simulink model "Model_OnlyDark_17_01_16"  (R2015a)
settings: Solver=FixedStepDiscrete  StartTime=0.0  StopTime=60  FixedStep=0.05  RelTol=1e-3
InitFcn:
  | %Ts=parameter.Ts;
  |    %Sampling Time, 50 times slower than original model
model workspace (MAT data in the model file):
  TimeStep = 0.05
  padsize = 8
  x1 = 14
  pixPR = 12
  hdegs = 90
  vdegs = 20
undefined symbols (not defined in the file): alpha_downslope_off, alpha_downslope_on, alpha_upslope_off, alpha_upslope_on, fdsr_lp
libraries: visionfilter x3, visionutilities x3
settings Model: tstep=0.1  TimeStep=0.1  CovSFcnEnable=off  Creator=a1174239  LastModifiedBy=John
settings SolverCC: AlgebraicLoopSolver=LineSearch
settings DataIOCC: MaxDataPoints=1
settings OptimizationCC: ExpressionDepthLimit=2147483647  EfficientMapNaN2IntZero=off
settings DebuggingCC: UnderspecifiedInitializationDetection=Classic  MergeDetectMultiDrivingBlocksExec=none  SolverPrmCheckMsg=warning  MultiTaskDSMMsg=warning  MultiTaskCondExecSysMsg=none  ParameterPrecisionLossMsg=none  StateNameClashWarn=warning
settings HardwareCC: TargetLongLongMode=on  TargetIntDivRoundTo=Zero  TargetEndianess=LittleEndian  TargetHWDeviceType=MATLAB Host  ProdEqTarget=off
settings CodeAppCC: MaxIdLength=128
settings GRTTargetCC: CombineOutputUpdateFcns=off  GRTInterface=on

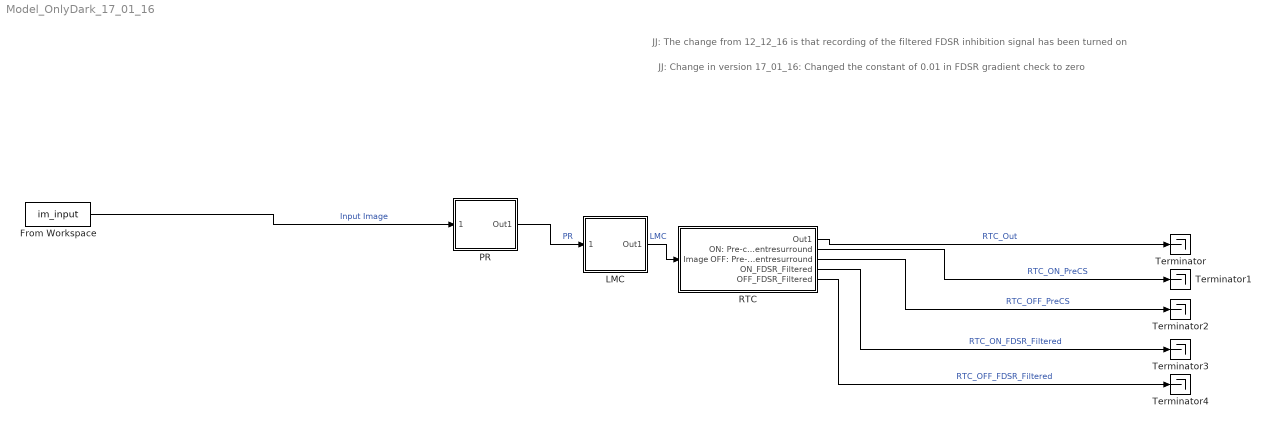
== system Model_OnlyDark_17_01_16 ==
  note: JJ: Change in version 17_01_16: Changed the constant of 0.01 in FDSR gradient check to zero
  note: JJ: The change from 12_12_16 is that recording of the filtered FDSR inhibition signal has been turned on
  From Workspace : FromWorkspace  VariableName=im_input  SampleTime=0.001  Interpolate=off  OutputAfterFinalValue=Holding final value
  LMC : Subsystem
  PR : Subsystem
  RTC : Subsystem
  Terminator{,1..4} (5 alike) : Terminator
  wires:
  PR/1(Out1) -> LMC/1(Image)  "PR"
  LMC/1(Out1) -> RTC/1(Image)  "LMC"
  RTC/1(Out1) -> Terminator/1  "RTC_Out"
  From Workspace/1 -> PR/1(Image)  "Input Image"
  RTC/2(ON: Pre-centresurround) -> Terminator1/1  "RTC_ON_PreCS"
  RTC/3(OFF: Pre-centresurround) -> Terminator2/1  "RTC_OFF_PreCS"
  RTC/4(ON_FDSR_Filtered) -> Terminator3/1  "RTC_ON_FDSR_Filtered"
  RTC/5(OFF_FDSR_Filtered) -> Terminator4/1  "RTC_OFF_FDSR_Filtered"

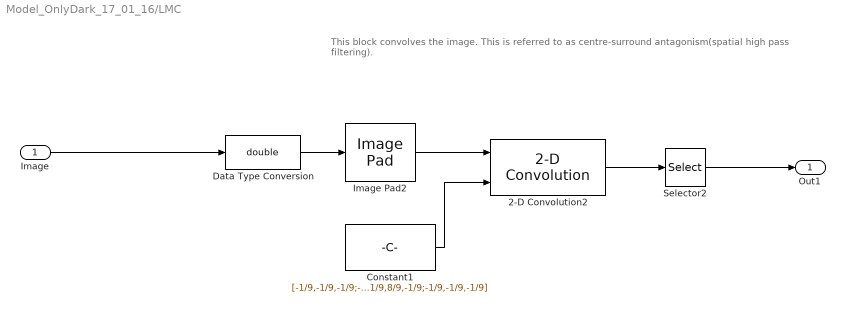
== system Model_OnlyDark_17_01_16/LMC ==
  note: This block convolves the image. This is referred to as centre-surround antagonism(spatial high pass filtering).
  Image : Inport
  2-D Convolution2 : visionfilter/2-D Convolution  outSize=Same as input port I1  normalize=off  outputMode=Binary point scaling  outputWordLength=32  outputFracLength=12  prodOutputMode=Binary point scaling  prodOutputWordLength=32  prodOutputFracLength=10  roundingMode=Floor  overflowMode=off
  Constant1 : Constant  Value=[-1/9,-1/9,-1/9;-1/9,8/9,-1/9;-1/9,-1/9,-1/9]
  Data Type Conversion : DataTypeConversion  OutDataTypeStr=double
  Image Pad2 : visionutilities/Image Pad  method=Symmetric  valSrc=Specify via dialog  value=0  spec=Pad size  rowDirection=Both left and right  outRowsMode=User-specified  rowSize=1  outColSize=10  colDirection=Both top and bottom  outColsMode=User-specified  colSize=1  outRowSize=12  trunc_flag=None
  Selector2 : Selector  NumberOfDimensions=2  InputPortWidth=3  IndexOptions=Index vector (dialog),Index vector (dialog)  Indices=[2:vdegs+1],[2:hdegs+1]  OutputSizes=1,1
  Out1 : Outport
  wires:
  Constant1/1 -> 2-D Convolution2/2
  Image Pad2/1 -> 2-D Convolution2/1
  2-D Convolution2/1 -> Selector2/1
  Selector2/1 -> Out1/1
  Image/1 -> Data Type Conversion/1
  Data Type Conversion/1 -> Image Pad2/1

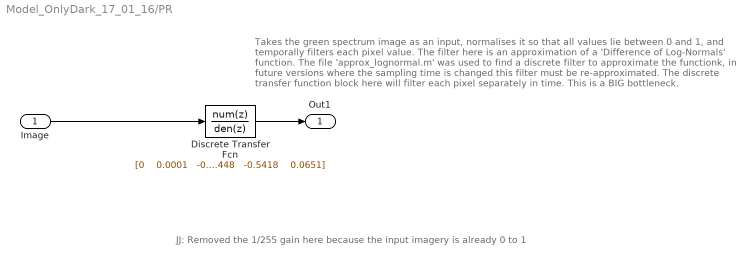
== system Model_OnlyDark_17_01_16/PR ==
  note: JJ: Removed the 1/255 gain here because the input imagery is already 0 to 1
  note: Takes the green spectrum image as an input, normalises it so that all values lie between 0
      | and 1, and temporally filters each pixel value. The filter here is an approximation of a
      | 'Difference of Log-Normals' function. The file 'approx_lognormal.m' was used to find a discrete
      | filter to approximate the functionk, in future versions where the sampling time is changed this filter
      | must be re-approximated.
      |
      | The discrete transfer function block here will filter each pixel separately in time. This is a BIG bottleneck.
  Image : Inport
  Discrete Transfer Fcn : DiscreteTransferFcn  Numerator="[0    0.0001   -0.0011    0.0052   -0.0170    0.0439   -0.0574    0.1789   -0.1524]"  Denominator="[ 1.0000   -4.3331    8.6847  -10.7116    9.0004   -5.3058    2.1448   -0.5418    0.0651]"
  Out1 : Outport
  wires:
  Image/1 -> Discrete Transfer Fcn/1
  Discrete Transfer Fcn/1 -> Out1/1

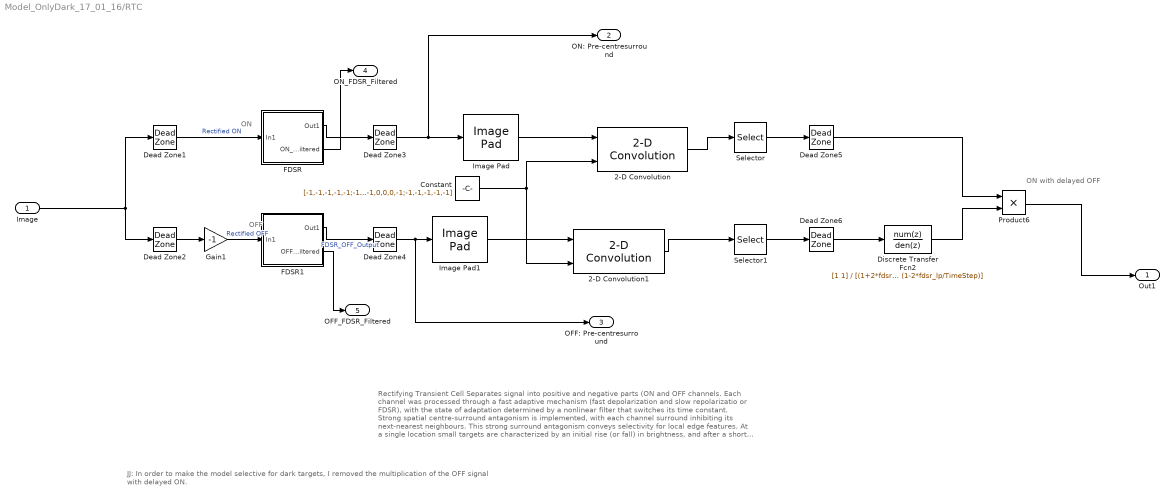
== system Model_OnlyDark_17_01_16/RTC ==
  note: ON with delayed OFF
  note: JJ: In order to make the model selective for dark targets, I removed the multiplication of the OFF signal with delayed ON.
  note: ON
  note: OFF
  note: Rectifying Transient Cell Separates signal into positive and negative parts (ON and OFF channels. Each channel was processed through a fast adaptive mechanism (fast depolarization and slow repolarizatio or FDSR),
      | with the state of adaptation determined by a nonlinear filter that switches its time constant. Strong spatial centre-surround antagonism is implemented, with each channel surround inhibiting its next-nearest neighbours.
      | This strong surround antagonism conveys selectivity for local edge features. At a single location small targets are characterized by an initial rise (or fall) in brightness, and after a short delay are followed by a corresponding
      | fall (or rise), irrespective of the direction of travel. Sensitivity to targets independent of their polarity was provided by multiplying each contrast channel (ON or OFF) with a delayed version of the opposite polarity
      | (via a low-pass filter,) and then summing the outputs.
  Image : Inport
  2-D Convolution : visionfilter/2-D Convolution  outSize=Same as input port I1  normalize=off  outputMode=Binary point scaling  outputWordLength=32  outputFracLength=12  prodOutputMode=Binary point scaling  prodOutputWordLength=32  prodOutputFracLength=10  roundingMode=Floor  overflowMode=off
  2-D Convolution1 : visionfilter/2-D Convolution  outSize=Same as input port I1  normalize=off  outputMode=Binary point scaling  outputWordLength=32  outputFracLength=12  prodOutputMode=Binary point scaling  prodOutputWordLength=32  prodOutputFracLength=10  roundingMode=Floor  overflowMode=off
  Constant : Constant  Value=[-1,-1,-1,-1,-1;-1,0,0,0,-1;-1,0,2,0,-1; -1,0,0,0,-1;-1,-1,-1,-1,-1]
  Dead Zone{1,3..6} (5 alike) : DeadZone  LowerValue=-inf  UpperValue=0  SaturateOnIntegerOverflow=on
  Dead Zone2 : DeadZone  LowerValue=0  UpperValue=inf  SaturateOnIntegerOverflow=on
  Discrete Transfer Fcn2 : DiscreteTransferFcn  Numerator=[1 1]  Denominator=[(1+2*fdsr_lp/TimeStep), (1-2*fdsr_lp/TimeStep)]
  FDSR : Subsystem
  FDSR1 : Subsystem
  Gain1 : Gain  Gain=-1
  Image Pad : visionutilities/Image Pad  method=Symmetric  valSrc=Specify via dialog  value=0  spec=Pad size  rowDirection=Both left and right  outRowsMode=User-specified  rowSize=2  outColSize=10  colDirection=Both top and bottom  outColsMode=User-specified  colSize=2  outRowSize=12  trunc_flag=None
  Image Pad1 : visionutilities/Image Pad  method=Symmetric  valSrc=Specify via dialog  value=0  spec=Pad size  rowDirection=Both left and right  outRowsMode=User-specified  rowSize=2  outColSize=10  colDirection=Both top and bottom  outColsMode=User-specified  colSize=2  outRowSize=12  trunc_flag=None
  Product6 : Product  RndMeth=Zero
  Selector : Selector  NumberOfDimensions=2  InputPortWidth=3  IndexOptions=Index vector (dialog),Index vector (dialog)  Indices=[3:vdegs+2],[3:hdegs+2]  OutputSizes=1,1
  Selector1 : Selector  NumberOfDimensions=2  InputPortWidth=3  IndexOptions=Index vector (dialog),Index vector (dialog)  Indices=[3:vdegs+2],[3:hdegs+2]  OutputSizes=1,1
  Out1 : Outport
  ON: Pre-centresurround : Outport  Port=2
  OFF: Pre-centresurround : Outport  Port=3
  ON_FDSR_Filtered : Outport  Port=4
  OFF_FDSR_Filtered : Outport  Port=5
  wires:
  Gain1/1 -> FDSR1/1(In1)  "Rectified OFF"
  Discrete Transfer Fcn2/1 -> Product6/2
  Dead Zone1/1 -> FDSR/1(In1)  "Rectified ON"
  Dead Zone2/1 -> Gain1/1
  FDSR/1(Out1) -> Dead Zone3/1
  FDSR1/1(Out1) -> Dead Zone4/1  "FDSR_OFF_Output"
  Image/1 -> Dead Zone1/1, Dead Zone2/1
  Dead Zone6/1 -> Discrete Transfer Fcn2/1
  Dead Zone5/1 -> Product6/1
  Image Pad/1 -> 2-D Convolution/1
  Constant/1 -> 2-D Convolution1/2, 2-D Convolution/2
  2-D Convolution/1 -> Selector/1
  Image Pad1/1 -> 2-D Convolution1/1
  2-D Convolution1/1 -> Selector1/1
  Dead Zone4/1 -> OFF: Pre-centresurround/1, Image Pad1/1
  Dead Zone3/1 -> ON: Pre-centresurround/1, Image Pad/1
  Selector1/1 -> Dead Zone6/1
  Selector/1 -> Dead Zone5/1
  FDSR1/2(OFF_FDSR_Filtered) -> OFF_FDSR_Filtered/1
  FDSR/2(ON_FDSR_Filtered) -> ON_FDSR_Filtered/1
  Product6/1 -> Out1/1

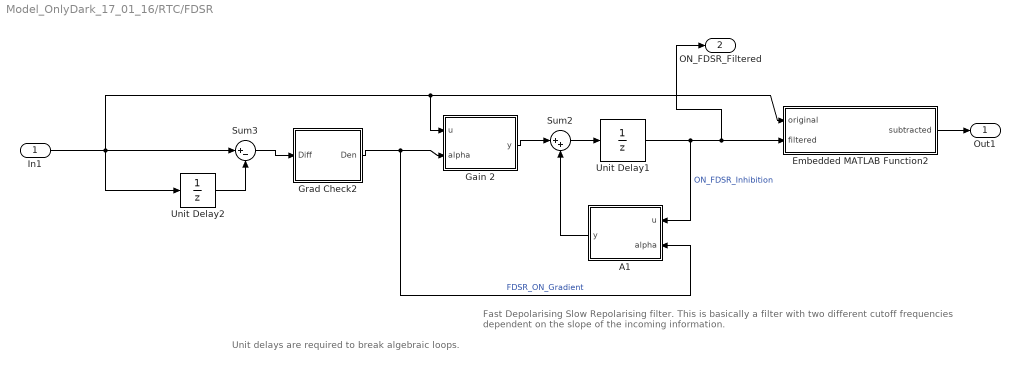
== system Model_OnlyDark_17_01_16/RTC/FDSR ==
  note: Fast Depolarising Slow Repolarising filter. This is basically a filter with two different cutoff frequencies dependent on the slope of the incoming information.
  note: Unit delays are required to break algebraic loops.
  In1 : Inport
  A1 : MATLAB Function  TreatAsAtomicUnit=on
  Embedded MATLAB Function2 : MATLAB Function  TreatAsAtomicUnit=on
  Gain 2 : MATLAB Function  TreatAsAtomicUnit=on
  Grad Check2 : Subsystem
  Sum2 : Sum  Inputs=|++
  Sum3 : Sum  Inputs=|+-
  Unit Delay1 : UnitDelay  SampleTime=-1
  Unit Delay2 : UnitDelay  SampleTime=-1
  Out1 : Outport
  ON_FDSR_Filtered : Outport  Port=2
  wires:
  Sum2/1 -> Unit Delay1/1
  Unit Delay1/1 -> A1/1(u), ON_FDSR_Filtered/1, Embedded MATLAB Function2/2(filtered)  "ON_FDSR_Inhibition"
  A1/1(y) -> Sum2/2
  Gain 2/1(y) -> Sum2/1
  In1/1 -> Unit Delay2/1, Sum3/1, Gain 2/1(u), Embedded MATLAB Function2/1(original)
  Unit Delay2/1 -> Sum3/2
  Sum3/1 -> Grad Check2/1(Diff)
  Grad Check2/1(Den) -> Gain 2/2(alpha), A1/2(alpha)  "FDSR_ON_Gradient"
  Embedded MATLAB Function2/1(subtracted) -> Out1/1

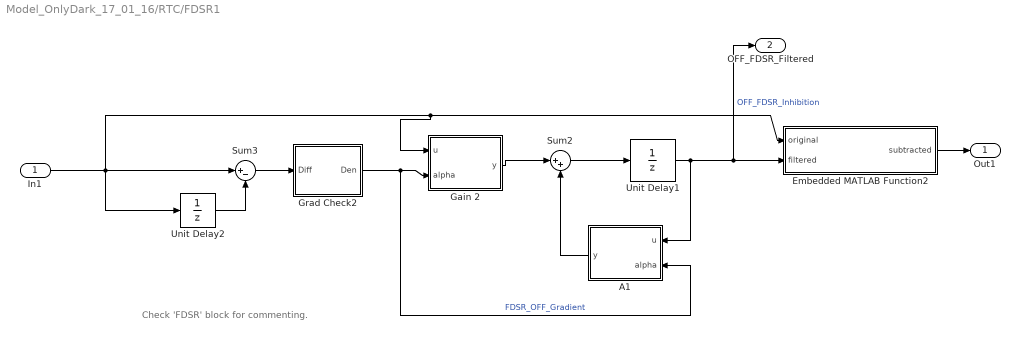
== system Model_OnlyDark_17_01_16/RTC/FDSR1 ==
  note: Check 'FDSR' block for commenting.
  In1 : Inport
  A1 : MATLAB Function  TreatAsAtomicUnit=on
  Embedded MATLAB Function2 : MATLAB Function  TreatAsAtomicUnit=on
  Gain 2 : MATLAB Function  TreatAsAtomicUnit=on
  Grad Check2 : Subsystem
  Sum2 : Sum  Inputs=|++
  Sum3 : Sum  Inputs=|+-
  Unit Delay1 : UnitDelay  SampleTime=-1
  Unit Delay2 : UnitDelay  SampleTime=-1
  Out1 : Outport
  OFF_FDSR_Filtered : Outport  Port=2
  wires:
  Embedded MATLAB Function2/1(subtracted) -> Out1/1
  Grad Check2/1(Den) -> A1/2(alpha), Gain 2/2(alpha)  "FDSR_OFF_Gradient"
  Sum3/1 -> Grad Check2/1(Diff)
  Unit Delay2/1 -> Sum3/2
  In1/1 -> Embedded MATLAB Function2/1(original), Gain 2/1(u), Sum3/1, Unit Delay2/1
  Gain 2/1(y) -> Sum2/1
  A1/1(y) -> Sum2/2
  Unit Delay1/1 -> OFF_FDSR_Filtered/1, Embedded MATLAB Function2/2(filtered), A1/1(u)  "OFF_FDSR_Inhibition"
  Sum2/1 -> Unit Delay1/1

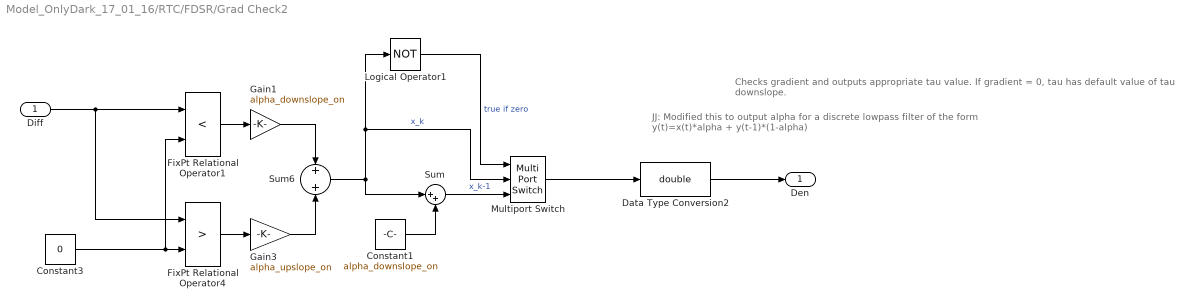
== system Model_OnlyDark_17_01_16/RTC/FDSR/Grad Check2 ==
  note: JJ: Modified this to output alpha for a discrete lowpass filter of the form
      | y(t)=x(t)*alpha + y(t-1)*(1-alpha)
  note: Checks gradient and outputs appropriate tau value. If gradient = 0, tau has default value of tau downslope.
  Diff : Inport
  Constant1 : Constant  Value=alpha_downslope_on
  Constant3 : Constant  Value=0
  Data Type Conversion2 : DataTypeConversion  OutDataTypeStr=double
  FixPt Relational Operator1 : RelationalOperator  Operator=<  OutDataTypeStr=fixdt(0, 8)  ZeroCross=off
  FixPt Relational Operator4 : RelationalOperator  Operator=>  OutDataTypeStr=fixdt(0, 8)  ZeroCross=off
  Gain1 : Gain  Gain=alpha_downslope_on
  Gain3 : Gain  Gain=alpha_upslope_on
  Logical Operator1 : Logic  Operator=NOT  AllPortsSameDT=off  OutDataTypeStr=boolean
  Multiport Switch : MultiPortSwitch  DataPortOrder=Zero-based contiguous  Inputs=2  zeroidx=on
  Sum : Sum  Inputs=|++
  Sum6 : Sum  Inputs=+|+
  Den : Outport
  wires:
  FixPt Relational Operator4/1 -> Gain3/1
  Gain1/1 -> Sum6/1
  Gain3/1 -> Sum6/2
  FixPt Relational Operator1/1 -> Gain1/1
  Constant3/1 -> FixPt Relational Operator1/2, FixPt Relational Operator4/2
  Diff/1 -> FixPt Relational Operator4/1, FixPt Relational Operator1/1
  Logical Operator1/1 -> Multiport Switch/1  "true if zero"
  Sum6/1 -> Logical Operator1/1, Multiport Switch/2, Sum/1  "x_k"
  Sum/1 -> Multiport Switch/3  "x_k-1"
  Data Type Conversion2/1 -> Den/1
  Multiport Switch/1 -> Data Type Conversion2/1
  Constant1/1 -> Sum/2

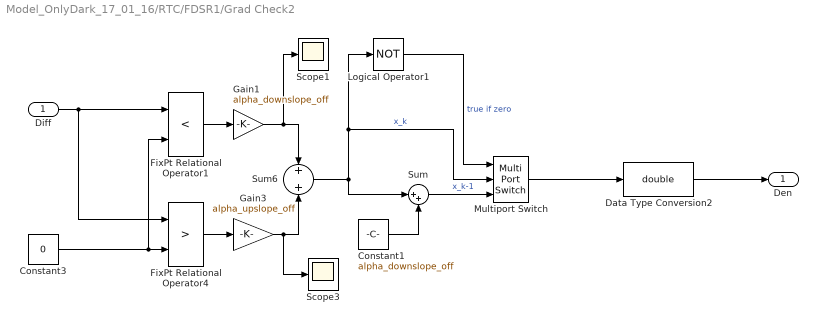
== system Model_OnlyDark_17_01_16/RTC/FDSR1/Grad Check2 ==
  Diff : Inport
  Constant1 : Constant  Value=alpha_downslope_off
  Constant3 : Constant  Value=0
  Data Type Conversion2 : DataTypeConversion  OutDataTypeStr=double
  FixPt Relational Operator1 : RelationalOperator  Operator=<  OutDataTypeStr=fixdt(0, 8)  ZeroCross=off
  FixPt Relational Operator4 : RelationalOperator  Operator=>  OutDataTypeStr=fixdt(0, 8)  ZeroCross=off
  Gain1 : Gain  Gain=alpha_downslope_off
  Gain3 : Gain  Gain=alpha_upslope_off
  Logical Operator1 : Logic  Operator=NOT  AllPortsSameDT=off  OutDataTypeStr=boolean
  Multiport Switch : MultiPortSwitch  DataPortOrder=Zero-based contiguous  Inputs=2  zeroidx=on
  Scope1 : Scope
      settings: SaveName=ScopeData5
  Scope3 : Scope
  Sum : Sum  Inputs=|++
  Sum6 : Sum  Inputs=+|+
  Den : Outport
  wires:
  Constant1/1 -> Sum/2
  Multiport Switch/1 -> Data Type Conversion2/1
  Data Type Conversion2/1 -> Den/1
  Sum/1 -> Multiport Switch/3  "x_k-1"
  Sum6/1 -> Sum/1, Multiport Switch/2, Logical Operator1/1  "x_k"
  Logical Operator1/1 -> Multiport Switch/1  "true if zero"
  Diff/1 -> FixPt Relational Operator1/1, FixPt Relational Operator4/1
  Constant3/1 -> FixPt Relational Operator4/2, FixPt Relational Operator1/2
  FixPt Relational Operator1/1 -> Gain1/1
  Gain3/1 -> Sum6/2, Scope3/1
  Gain1/1 -> Scope1/1, Sum6/1
  FixPt Relational Operator4/1 -> Gain3/1

== matlab function Model_OnlyDark_17_01_16/RTC/FDSR/A1 ==
  data: u input; y output; alpha input
function y = fcn(u, alpha)
%#eml

y=(1-alpha).*u;
% Previous version below. Gradient check used to output tau.
%y = (exp(-(Ts./tau))).*u;

== matlab function Model_OnlyDark_17_01_16/RTC/FDSR1/A1 ==
  data: u input; y output; alpha input
function y = fcn(u, alpha)
%#eml

y=u.*(1-alpha);

%Old way below
%y = (exp(-(Ts./tau))).*u;

== matlab function Model_OnlyDark_17_01_16/RTC/FDSR/Gain 2 ==
  data: u input; y output; alpha input
function y = fcn(u, alpha)
%#eml
y=u.*alpha;

%Below is the previous version. Note that prior to the change, the gradient
%check block outputted tau.
%y = (1-exp(-(Ts./tau))).*u;

== matlab function Model_OnlyDark_17_01_16/RTC/FDSR/Embedded MATLAB Function2 ==
  data: original input; filtered input; subtracted output
% for some strange reason the code doesnt like normal 'subtract' blocks
% right here, so an embedded function block was used instead. Just another one of
% MATLABs random errors.

function subtracted = subtract(original, filtered)
%#eml

subtracted = original-filtered;

== matlab function Model_OnlyDark_17_01_16/RTC/FDSR1/Embedded MATLAB Function2 ==
  data: original input; filtered input; subtracted output
function subtracted = subtract(original, filtered)
%#eml

subtracted = original-filtered;

== matlab function Model_OnlyDark_17_01_16/RTC/FDSR1/Gain 2 ==
  data: u input; y output; alpha input
function y = fcn(u, alpha)
%#eml

y=u.*alpha;

%Below is the old way of calculating this
%y = (1-exp(-(Ts./tau))).*u;
